simulink library "dfr_id"  (Simulink 8.1)
settings: Solver=ode1  StartTime=0.0  StopTime=Inf  FixedStep=0.001  RelTol=1e-3
PostLoadFcn:
  | , if any(exist('dsrtsu_mdlpostloadfcn', 'file') == [2, 3, 6]), try dsrtsu_mdlpostloadfcn('Execute', bdroot); catch fprintf('Error in PostLoadFcn (dsrtsu_mdlpostloadfcn) for model "%s":\n %s\n', bdroot, lasterr); end, end,
undefined symbols (not defined in the file or in its folder): ENUM_PMMSTATE_NORMAL, FALSE, TRUE, ZERO_FLOAT, ZERO_INT
settings Model: DSRTSU_INTERNAL_RTI_VER=450  DSRTSU_INTERNAL_RTI_TYPE=rti1401  RTICANMMDATA=struct('GeneralSetupData',struct('modelroot','D:\ELN150201\Phase3\trunk\Application\AdasDragon\software\sw_development\arch\app\dfr','generalsettings',struct('filesettings',struct('destfolder',struct('Name','RTICANMM_FILES','Check',1),'buildfolder',struct('Name','.','Check',1),'AbsDestfolder',struct('Name','D:\ELN150201\Phase3\trunk\Application\AdasDragon\software\sw_development\arch\app\dfr\RTICANMM_FILES'),'AbsBuildfolder',struct('Name','D:\ELN150201\Phase3\trunk\Application\AdasDragon\software\sw_development\arch\app\dfr'))),'options',struct('addpaths',1,'rmpaths',1,'addtrcexclusion',logical(1),'cannavigator',struct('checkmonitoring',0),'show_usrtrc',0,'use_usrtrc',0),'advanced',struct('options',[1 1 1 1 1 1 1 1 1 1 1 1 1 1 1 1 1 1 1 1 1 1 1 1 1 1 1 1 1 1 1 1 1 1 1 1 1 1 1 1 1 1 1 1 1 1 1 1 1 1 1 1 1 1 1 1 1 1 1 1 1 1 1 1 1 1 1 1 1 1 1 1 1 1 1 1 1 1 1 1 1 1 1 1 1 1 1 1 1 1 1 1 1 1 1 1 1 1 1 1]),'MPSetup',{{}},'modelname','dfr_id','block','dfr_id'))  DSRTSU_INTERNAL_RTIFPGA=40  Creator=tescamilla  LastModifiedBy=AT015555

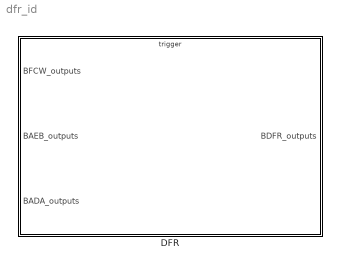
== system dfr_id ==
  DFR : Subsystem
      settings: RTWSystemCode=Nonreusable function  RTWFcnNameOpts=Use subsystem name  RTWFileNameOpts=Use subsystem name

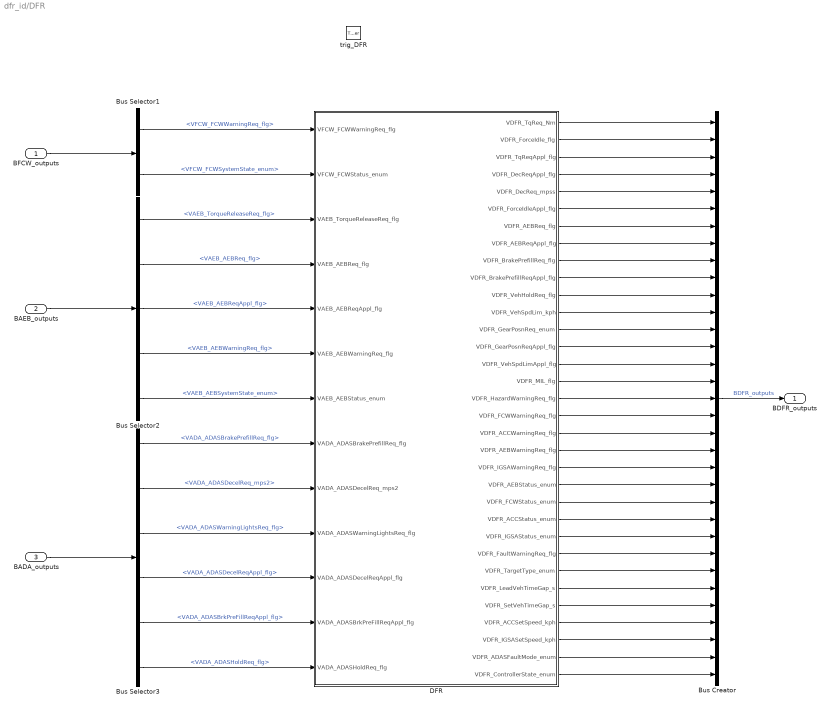
== system dfr_id/DFR ==
  BFCW_outputs : Inport  OutDataTypeStr=Bus: BFCW_outputs
  BAEB_outputs : Inport  Port=2  OutDataTypeStr=Bus: BAEB_outputs
  BADA_outputs : Inport  Port=3  OutDataTypeStr=Bus: BADA_outputs
  trig_DFR : TriggerPort  TriggerType=function-call
  Bus Creator : BusCreator  Inputs=33  OutDataTypeStr=Bus: BDFR_outputs
  Bus Selector1 : BusSelector  OutputSignals=VFCW_FCWWarningReq_flg,VFCW_FCWSystemState_enum
  Bus Selector2 : BusSelector  OutputSignals=VAEB_TorqueReleaseReq_flg,VAEB_AEBReq_flg,VAEB_AEBReqAppl_flg,VAEB_AEBWarningReq_flg,VAEB_AEBSystemState_enum
  Bus Selector3 : BusSelector  OutputSignals=VADA_ADASBrakePrefillReq_flg,VADA_ADASDecelReq_mps2,VADA_ADASWarningLightsReq_flg,VADA_ADASDecelReqAppl_flg,VADA_ADASBrkPreFillReqAppl_flg,VADA_ADASHoldReq_flg
  DFR : Subsystem
  BDFR_outputs : Outport  OutDataTypeStr=Bus: BDFR_outputs
  wires:
  DFR/33(VDFR_ControllerState_enum) -> Bus Creator/33
  Bus Selector1/1 -> DFR/1(VFCW_FCWWarningReq_flg)  "<VFCW_FCWWarningReq_flg>"
  DFR/1(VDFR_TqReq_Nm) -> Bus Creator/1
  DFR/31(VDFR_IGSASetSpeed_kph) -> Bus Creator/31
  DFR/11(VDFR_VehHoldReq_flg) -> Bus Creator/11
  DFR/14(VDFR_GearPosnReqAppl_flg) -> Bus Creator/14
  DFR/32(VDFR_ADASFaultMode_enum) -> Bus Creator/32
  DFR/17(VDFR_HazardWarningReq_flg) -> Bus Creator/17
  DFR/13(VDFR_GearPosnReq_enum) -> Bus Creator/13
  DFR/19(VDFR_ACCWarningReq_flg) -> Bus Creator/19
  DFR/16(VDFR_MIL_flg) -> Bus Creator/16
  DFR/15(VDFR_VehSpdLimAppl_flg) -> Bus Creator/15
  DFR/20(VDFR_AEBWarningReq_flg) -> Bus Creator/20
  DFR/12(VDFR_VehSpdLim_kph) -> Bus Creator/12
  DFR/18(VDFR_FCWWarningReq_flg) -> Bus Creator/18
  DFR/23(VDFR_FCWStatus_enum) -> Bus Creator/23
  DFR/22(VDFR_AEBStatus_enum) -> Bus Creator/22
  DFR/30(VDFR_ACCSetSpeed_kph) -> Bus Creator/30
  DFR/24(VDFR_ACCStatus_enum) -> Bus Creator/24
  DFR/26(VDFR_FaultWarningReq_flg) -> Bus Creator/26
  DFR/28(VDFR_LeadVehTimeGap_s) -> Bus Creator/28
  DFR/21(VDFR_IGSAWarningReq_flg) -> Bus Creator/21
  DFR/29(VDFR_SetVehTimeGap_s) -> Bus Creator/29
  DFR/27(VDFR_TargetType_enum) -> Bus Creator/27
  DFR/25(VDFR_IGSAStatus_enum) -> Bus Creator/25
  DFR/7(VDFR_AEBReq_flg) -> Bus Creator/7
  DFR/8(VDFR_AEBReqAppl_flg) -> Bus Creator/8
  DFR/4(VDFR_DecReqAppl_flg) -> Bus Creator/4
  DFR/5(VDFR_DecReq_mpss) -> Bus Creator/5
  DFR/6(VDFR_ForceIdleAppl_flg) -> Bus Creator/6
  DFR/3(VDFR_TqReqAppl_flg) -> Bus Creator/3
  DFR/10(VDFR_BrakePrefillReqAppl_flg) -> Bus Creator/10
  DFR/9(VDFR_BrakePrefillReq_flg) -> Bus Creator/9
  DFR/2(VDFR_ForceIdle_flg) -> Bus Creator/2
  Bus Selector1/2 -> DFR/2(VFCW_FCWStatus_enum)  "<VFCW_FCWSystemState_enum>"
  Bus Creator/1 -> BDFR_outputs/1  "BDFR_outputs"
  BFCW_outputs/1 -> Bus Selector1/1
  BAEB_outputs/1 -> Bus Selector2/1
  Bus Selector2/4 -> DFR/6(VAEB_AEBWarningReq_flg)  "<VAEB_AEBWarningReq_flg>"
  Bus Selector2/5 -> DFR/7(VAEB_AEBStatus_enum)  "<VAEB_AEBSystemState_enum>"
  Bus Selector2/3 -> DFR/5(VAEB_AEBReqAppl_flg)  "<VAEB_AEBReqAppl_flg>"
  Bus Selector2/2 -> DFR/4(VAEB_AEBReq_flg)  "<VAEB_AEBReq_flg>"
  Bus Selector2/1 -> DFR/3(VAEB_TorqueReleaseReq_flg)  "<VAEB_TorqueReleaseReq_flg>"
  BADA_outputs/1 -> Bus Selector3/1
  Bus Selector3/6 -> DFR/13(VADA_ADASHoldReq_flg)  "<VADA_ADASHoldReq_flg>"
  Bus Selector3/1 -> DFR/8(VADA_ADASBrakePrefillReq_flg)  "<VADA_ADASBrakePrefillReq_flg>"
  Bus Selector3/2 -> DFR/9(VADA_ADASDecelReq_mps2)  "<VADA_ADASDecelReq_mps2>"
  Bus Selector3/3 -> DFR/10(VADA_ADASWarningLightsReq_flg)  "<VADA_ADASWarningLightsReq_flg>"
  Bus Selector3/4 -> DFR/11(VADA_ADASDecelReqAppl_flg)  "<VADA_ADASDecelReqAppl_flg>"
  Bus Selector3/5 -> DFR/12(VADA_ADASBrkPreFillReqAppl_flg)  "<VADA_ADASBrkPreFillReqAppl_flg>"

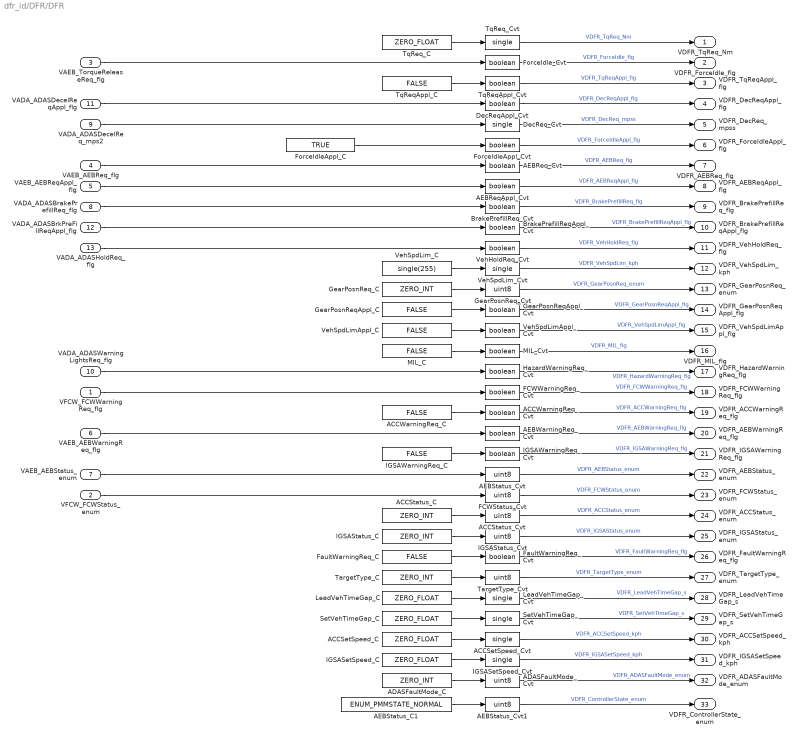
== system dfr_id/DFR/DFR ==
  VFCW_FCWWarningReq_flg : Inport
  VFCW_FCWStatus_enum : Inport  Port=2
  VAEB_TorqueReleaseReq_flg : Inport  Port=3
  VAEB_AEBReq_flg : Inport  Port=4
  VAEB_AEBReqAppl_flg : Inport  Port=5
  VAEB_AEBWarningReq_flg : Inport  Port=6
  VAEB_AEBStatus_enum : Inport  Port=7
  VADA_ADASBrakePrefillReq_flg : Inport  Port=8
  VADA_ADASDecelReq_mps2 : Inport  Port=9
  VADA_ADASWarningLightsReq_flg : Inport  Port=10
  VADA_ADASDecelReqAppl_flg : Inport  Port=11
  VADA_ADASBrkPreFillReqAppl_flg : Inport  Port=12
  VADA_ADASHoldReq_flg : Inport  Port=13
  ACCSetSpeed_C : Constant  Value=ZERO_FLOAT
  ACCSetSpeed_Cvt : DataTypeConversion  OutDataTypeStr=single  SaturateOnIntegerOverflow=on  RndMeth=Zero
  ACCStatus_C : Constant  Value=ZERO_INT
  ACCStatus_Cvt : DataTypeConversion  OutDataTypeStr=uint8  SaturateOnIntegerOverflow=on  RndMeth=Zero
  ACCWarningReq_C : Constant  Value=FALSE
  ACCWarningReq_Cvt : DataTypeConversion  OutDataTypeStr=boolean  SaturateOnIntegerOverflow=on  RndMeth=Zero
  ADASFaultMode_C : Constant  Value=ZERO_INT
  ADASFaultMode_Cvt : DataTypeConversion  OutDataTypeStr=uint8  SaturateOnIntegerOverflow=on  RndMeth=Zero
  AEBReqAppl_Cvt : DataTypeConversion  OutDataTypeStr=boolean  SaturateOnIntegerOverflow=on  RndMeth=Zero
  AEBReq_Cvt : DataTypeConversion  OutDataTypeStr=boolean  SaturateOnIntegerOverflow=on  RndMeth=Zero
  AEBStatus_C1 : Constant  Value=ENUM_PMMSTATE_NORMAL
  AEBStatus_Cvt : DataTypeConversion  OutDataTypeStr=uint8  SaturateOnIntegerOverflow=on  RndMeth=Zero
  AEBStatus_Cvt1 : DataTypeConversion  OutDataTypeStr=uint8  SaturateOnIntegerOverflow=on  RndMeth=Zero
  AEBWarningReq_Cvt : DataTypeConversion  OutDataTypeStr=boolean  SaturateOnIntegerOverflow=on  RndMeth=Zero
  BrakePrefillReqAppl_Cvt : DataTypeConversion  OutDataTypeStr=boolean  SaturateOnIntegerOverflow=on  RndMeth=Zero
  BrakePrefillReq_Cvt : DataTypeConversion  OutDataTypeStr=boolean  SaturateOnIntegerOverflow=on  RndMeth=Zero
  DecReqAppl_Cvt : DataTypeConversion  OutDataTypeStr=boolean  SaturateOnIntegerOverflow=on  RndMeth=Zero
  DecReq_Cvt : DataTypeConversion  OutDataTypeStr=single  SaturateOnIntegerOverflow=on  RndMeth=Zero
  FCWStatus_Cvt : DataTypeConversion  OutDataTypeStr=uint8  SaturateOnIntegerOverflow=on  RndMeth=Zero
  FCWWarningReq_Cvt : DataTypeConversion  OutDataTypeStr=boolean  SaturateOnIntegerOverflow=on  RndMeth=Zero
  FaultWarningReq_C : Constant  Value=FALSE
  FaultWarningReq_Cvt : DataTypeConversion  OutDataTypeStr=boolean  SaturateOnIntegerOverflow=on  RndMeth=Zero
  ForceIdleAppl_C : Constant  Value=TRUE
  ForceIdleAppl_Cvt : DataTypeConversion  OutDataTypeStr=boolean  SaturateOnIntegerOverflow=on  RndMeth=Zero
  ForceIdle_Cvt : DataTypeConversion  OutDataTypeStr=boolean  SaturateOnIntegerOverflow=on  RndMeth=Zero
  GearPosnReqAppl_C : Constant  Value=FALSE
  GearPosnReqAppl_Cvt : DataTypeConversion  OutDataTypeStr=boolean  SaturateOnIntegerOverflow=on  RndMeth=Zero
  GearPosnReq_C : Constant  Value=ZERO_INT
  GearPosnReq_Cvt : DataTypeConversion  OutDataTypeStr=uint8  SaturateOnIntegerOverflow=on  RndMeth=Zero
  HazardWarningReq_Cvt : DataTypeConversion  OutDataTypeStr=boolean  SaturateOnIntegerOverflow=on  RndMeth=Zero
  IGSASetSpeed_C : Constant  Value=ZERO_FLOAT
  IGSASetSpeed_Cvt : DataTypeConversion  OutDataTypeStr=single  SaturateOnIntegerOverflow=on  RndMeth=Zero
  IGSAStatus_C : Constant  Value=ZERO_INT
  IGSAStatus_Cvt : DataTypeConversion  OutDataTypeStr=uint8  SaturateOnIntegerOverflow=on  RndMeth=Zero
  IGSAWarningReq_C : Constant  Value=FALSE
  IGSAWarningReq_Cvt : DataTypeConversion  OutDataTypeStr=boolean  SaturateOnIntegerOverflow=on  RndMeth=Zero
  LeadVehTimeGap_C : Constant  Value=ZERO_FLOAT
  LeadVehTimeGap_Cvt : DataTypeConversion  OutDataTypeStr=single  SaturateOnIntegerOverflow=on  RndMeth=Zero
  MIL_C : Constant  Value=FALSE
  MIL_Cvt : DataTypeConversion  OutDataTypeStr=boolean  SaturateOnIntegerOverflow=on  RndMeth=Zero
  SetVehTimeGap_C : Constant  Value=ZERO_FLOAT
  SetVehTimeGap_Cvt : DataTypeConversion  OutDataTypeStr=single  SaturateOnIntegerOverflow=on  RndMeth=Zero
  TargetType_C : Constant  Value=ZERO_INT
  TargetType_Cvt : DataTypeConversion  OutDataTypeStr=uint8  SaturateOnIntegerOverflow=on  RndMeth=Zero
  TqReqAppl_C : Constant  Value=FALSE
  TqReqAppl_Cvt : DataTypeConversion  OutDataTypeStr=boolean  SaturateOnIntegerOverflow=on  RndMeth=Zero
  TqReq_C : Constant  Value=ZERO_FLOAT
  TqReq_Cvt : DataTypeConversion  OutDataTypeStr=single  SaturateOnIntegerOverflow=on  RndMeth=Zero
  VehHoldReq_Cvt : DataTypeConversion  OutDataTypeStr=boolean  SaturateOnIntegerOverflow=on  RndMeth=Zero
  VehSpdLimAppl_C : Constant  Value=FALSE
  VehSpdLimAppl_Cvt : DataTypeConversion  OutDataTypeStr=boolean  SaturateOnIntegerOverflow=on  RndMeth=Zero
  VehSpdLim_C : Constant  Value=single(255)
  VehSpdLim_Cvt : DataTypeConversion  OutDataTypeStr=single  SaturateOnIntegerOverflow=on  RndMeth=Zero
  VDFR_TqReq_Nm : Outport
  VDFR_ForceIdle_flg : Outport  Port=2
  VDFR_TqReqAppl_flg : Outport  Port=3
  VDFR_DecReqAppl_flg : Outport  Port=4
  VDFR_DecReq_mpss : Outport  Port=5
  VDFR_ForceIdleAppl_flg : Outport  Port=6
  VDFR_AEBReq_flg : Outport  Port=7
  VDFR_AEBReqAppl_flg : Outport  Port=8
  VDFR_BrakePrefillReq_flg : Outport  Port=9
  VDFR_BrakePrefillReqAppl_flg : Outport  Port=10
  VDFR_VehHoldReq_flg : Outport  Port=11
  VDFR_VehSpdLim_kph : Outport  Port=12
  VDFR_GearPosnReq_enum : Outport  Port=13
  VDFR_GearPosnReqAppl_flg : Outport  Port=14
  VDFR_VehSpdLimAppl_flg : Outport  Port=15
  VDFR_MIL_flg : Outport  Port=16
  VDFR_HazardWarningReq_flg : Outport  Port=17
  VDFR_FCWWarningReq_flg : Outport  Port=18
  VDFR_ACCWarningReq_flg : Outport  Port=19
  VDFR_AEBWarningReq_flg : Outport  Port=20
  VDFR_IGSAWarningReq_flg : Outport  Port=21
  VDFR_AEBStatus_enum : Outport  Port=22
  VDFR_FCWStatus_enum : Outport  Port=23
  VDFR_ACCStatus_enum : Outport  Port=24
  VDFR_IGSAStatus_enum : Outport  Port=25
  VDFR_FaultWarningReq_flg : Outport  Port=26
  VDFR_TargetType_enum : Outport  Port=27
  VDFR_LeadVehTimeGap_s : Outport  Port=28
  VDFR_SetVehTimeGap_s : Outport  Port=29
  VDFR_ACCSetSpeed_kph : Outport  Port=30
  VDFR_IGSASetSpeed_kph : Outport  Port=31
  VDFR_ADASFaultMode_enum : Outport  Port=32
  VDFR_ControllerState_enum : Outport  Port=33
  wires:
  AEBStatus_Cvt1/1 -> VDFR_ControllerState_enum/1  "VDFR_ControllerState_enum"
  AEBStatus_C1/1 -> AEBStatus_Cvt1/1
  ADASFaultMode_Cvt/1 -> VDFR_ADASFaultMode_enum/1  "VDFR_ADASFaultMode_enum"
  ADASFaultMode_C/1 -> ADASFaultMode_Cvt/1
  IGSASetSpeed_Cvt/1 -> VDFR_IGSASetSpeed_kph/1  "VDFR_IGSASetSpeed_kph"
  IGSASetSpeed_C/1 -> IGSASetSpeed_Cvt/1
  ACCSetSpeed_Cvt/1 -> VDFR_ACCSetSpeed_kph/1  "VDFR_ACCSetSpeed_kph"
  ACCSetSpeed_C/1 -> ACCSetSpeed_Cvt/1
  SetVehTimeGap_Cvt/1 -> VDFR_SetVehTimeGap_s/1  "VDFR_SetVehTimeGap_s"
  SetVehTimeGap_C/1 -> SetVehTimeGap_Cvt/1
  LeadVehTimeGap_Cvt/1 -> VDFR_LeadVehTimeGap_s/1  "VDFR_LeadVehTimeGap_s"
  LeadVehTimeGap_C/1 -> LeadVehTimeGap_Cvt/1
  TargetType_Cvt/1 -> VDFR_TargetType_enum/1  "VDFR_TargetType_enum"
  TargetType_C/1 -> TargetType_Cvt/1
  FaultWarningReq_Cvt/1 -> VDFR_FaultWarningReq_flg/1  "VDFR_FaultWarningReq_flg"
  FaultWarningReq_C/1 -> FaultWarningReq_Cvt/1
  IGSAStatus_Cvt/1 -> VDFR_IGSAStatus_enum/1  "VDFR_IGSAStatus_enum"
  IGSAStatus_C/1 -> IGSAStatus_Cvt/1
  ACCStatus_Cvt/1 -> VDFR_ACCStatus_enum/1  "VDFR_ACCStatus_enum"
  ACCStatus_C/1 -> ACCStatus_Cvt/1
  FCWStatus_Cvt/1 -> VDFR_FCWStatus_enum/1  "VDFR_FCWStatus_enum"
  VFCW_FCWStatus_enum/1 -> FCWStatus_Cvt/1
  AEBStatus_Cvt/1 -> VDFR_AEBStatus_enum/1  "VDFR_AEBStatus_enum"
  VAEB_AEBStatus_enum/1 -> AEBStatus_Cvt/1
  IGSAWarningReq_Cvt/1 -> VDFR_IGSAWarningReq_flg/1  "VDFR_IGSAWarningReq_flg"
  IGSAWarningReq_C/1 -> IGSAWarningReq_Cvt/1
  AEBWarningReq_Cvt/1 -> VDFR_AEBWarningReq_flg/1  "VDFR_AEBWarningReq_flg"
  VAEB_AEBWarningReq_flg/1 -> AEBWarningReq_Cvt/1
  ACCWarningReq_Cvt/1 -> VDFR_ACCWarningReq_flg/1  "VDFR_ACCWarningReq_flg"
  ACCWarningReq_C/1 -> ACCWarningReq_Cvt/1
  FCWWarningReq_Cvt/1 -> VDFR_FCWWarningReq_flg/1  "VDFR_FCWWarningReq_flg"
  VFCW_FCWWarningReq_flg/1 -> FCWWarningReq_Cvt/1
  HazardWarningReq_Cvt/1 -> VDFR_HazardWarningReq_flg/1  "VDFR_HazardWarningReq_flg"
  VADA_ADASWarningLightsReq_flg/1 -> HazardWarningReq_Cvt/1
  MIL_Cvt/1 -> VDFR_MIL_flg/1  "VDFR_MIL_flg"
  MIL_C/1 -> MIL_Cvt/1
  VehSpdLimAppl_Cvt/1 -> VDFR_VehSpdLimAppl_flg/1  "VDFR_VehSpdLimAppl_flg"
  VehSpdLimAppl_C/1 -> VehSpdLimAppl_Cvt/1
  GearPosnReqAppl_Cvt/1 -> VDFR_GearPosnReqAppl_flg/1  "VDFR_GearPosnReqAppl_flg"
  GearPosnReqAppl_C/1 -> GearPosnReqAppl_Cvt/1
  GearPosnReq_Cvt/1 -> VDFR_GearPosnReq_enum/1  "VDFR_GearPosnReq_enum"
  GearPosnReq_C/1 -> GearPosnReq_Cvt/1
  VehSpdLim_Cvt/1 -> VDFR_VehSpdLim_kph/1  "VDFR_VehSpdLim_kph"
  VehSpdLim_C/1 -> VehSpdLim_Cvt/1
  VehHoldReq_Cvt/1 -> VDFR_VehHoldReq_flg/1  "VDFR_VehHoldReq_flg"
  VADA_ADASHoldReq_flg/1 -> VehHoldReq_Cvt/1
  BrakePrefillReqAppl_Cvt/1 -> VDFR_BrakePrefillReqAppl_flg/1  "VDFR_BrakePrefillReqAppl_flg"
  VADA_ADASBrakePrefillReq_flg/1 -> BrakePrefillReq_Cvt/1
  BrakePrefillReq_Cvt/1 -> VDFR_BrakePrefillReq_flg/1  "VDFR_BrakePrefillReq_flg"
  AEBReqAppl_Cvt/1 -> VDFR_AEBReqAppl_flg/1  "VDFR_AEBReqAppl_flg"
  VAEB_AEBReqAppl_flg/1 -> AEBReqAppl_Cvt/1
  AEBReq_Cvt/1 -> VDFR_AEBReq_flg/1  "VDFR_AEBReq_flg"
  VAEB_AEBReq_flg/1 -> AEBReq_Cvt/1
  ForceIdleAppl_Cvt/1 -> VDFR_ForceIdleAppl_flg/1  "VDFR_ForceIdleAppl_flg"
  ForceIdleAppl_C/1 -> ForceIdleAppl_Cvt/1
  DecReq_Cvt/1 -> VDFR_DecReq_mpss/1  "VDFR_DecReq_mpss"
  VADA_ADASDecelReq_mps2/1 -> DecReq_Cvt/1
  DecReqAppl_Cvt/1 -> VDFR_DecReqAppl_flg/1  "VDFR_DecReqAppl_flg"
  VADA_ADASDecelReqAppl_flg/1 -> DecReqAppl_Cvt/1
  TqReqAppl_Cvt/1 -> VDFR_TqReqAppl_flg/1  "VDFR_TqReqAppl_flg"
  TqReqAppl_C/1 -> TqReqAppl_Cvt/1
  ForceIdle_Cvt/1 -> VDFR_ForceIdle_flg/1  "VDFR_ForceIdle_flg"
  VAEB_TorqueReleaseReq_flg/1 -> ForceIdle_Cvt/1
  TqReq_Cvt/1 -> VDFR_TqReq_Nm/1  "VDFR_TqReq_Nm"
  TqReq_C/1 -> TqReq_Cvt/1
  VADA_ADASBrkPreFillReqAppl_flg/1 -> BrakePrefillReqAppl_Cvt/1
